simulink model "test_of_write"  (R2020a)
settings: Solver=VariableStepAuto  StartTime=0.0  StopTime=inf  RelTol=1e-3
undefined symbols (not defined in the file or in its folder): requestFromServer, send2Server
libraries: realtime_pacer_lib x1
settings Model: Creator=Casper  LastModifiedBy=Casper

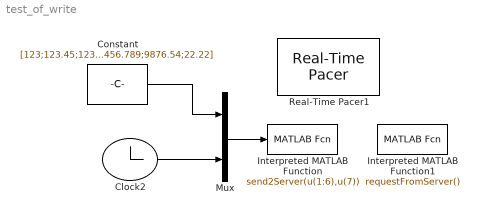
== system test_of_write ==
  Clock2 : Clock
      settings: Decimation=4
  Constant : Constant  Value=[123;123.45;12345.678;456.789;9876.54;22.22]
  Interpreted MATLAB Function : MATLABFcn  MATLABFcn=send2Server(u(1:6),u(7))  OutputDimensions=0
  Interpreted MATLAB Function1 : MATLABFcn  MATLABFcn=requestFromServer()  OutputDimensions=8
  Mux : Mux  Inputs=2
  Real-Time Pacer1 : realtime_pacer_lib/Real-Time Pacer  simTimePerRealTime=1
  wires:
  Clock2/1 -> Mux/2
  Constant/1 -> Mux/1
  Mux/1 -> Interpreted MATLAB Function/1
